simulink model "quad_mpc_nn_3_ref"  (R2020a)
settings: Solver=FixedStepAuto  StartTime=0.0  StopTime=20  FixedStep=0.01  RelTol=1e-3
values from neighbouring files (symbols this model uses):
  no_y = 6    [main_quad_mpc.m]
  x0 = [7;-10;0;0;0;0;0;0;0;0;0;0]    [main_quad_mpc.m]
libraries: neural x38
(part 3 of 3)

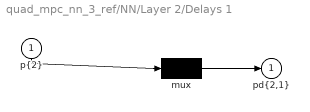
== system quad_mpc_nn_3_ref/NN/Layer 2/Delays 1 ==
  "p{2}" : Inport  PortDimensions=30
      mask Display: e = 0.06;c1 = [120 230 180]/255;c2 = ([120 230 180]+0)/(256+128);c3 = ([120 230 180]+128)/(256+128);patch([0 1 1 0],[0 0 1 1],c1);patch([0 1 1 1-e 1-e 0+e],[0 0 1 1-e 0+e 0+e],c2);patch([0 0 1 1-e 0+e 0+e],[0 1 1 1-e 1-e 0+e],c3);plot([0 1 1 0 0],[0 0 1 1 0]);
  mux : Mux  Inputs=1
      mask Display: e = 0.06;c1 = [120 150 230]/255;c2 = ([120 150 230]+0)/383;c3 = ([120 150 230]+128)/383;patch([0 1 1 0],[0 0 1 1],c1);patch([0 1 1 1-e 1-e 0+e],[0 0 1 1-e 0+e 0+e],c2);patch([0 0 1 1-e 0+e 0+e],[0 1 1 1-e 1-e 0+e],c3);plot([0 1 1 0 0],[0 0 1 1 0]);disp('Mux')
  "pd{2,1}" : Outport
      mask Display: e = 0.06;c1 = [120 230 180]/255;c2 = ([120 230 180]+0)/(256+128);c3 = ([120 230 180]+128)/(256+128);patch([0 1 1 0],[0 0 1 1],c1);patch([0 1 1 1-e 1-e 0+e],[0 0 1 1-e 0+e 0+e],c2);patch([0 0 1 1-e 0+e 0+e],[0 1 1 1-e 1-e 0+e],c3);plot([0 1 1 0 0],[0 0 1 1 0]);
  wires:
  "p{2}"/1 -> mux/1
  mux/1 -> "pd{2,1}"/1

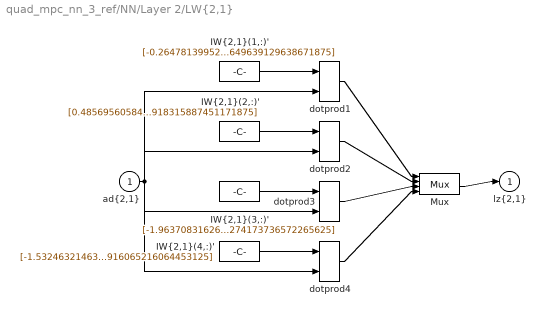
== system quad_mpc_nn_3_ref/NN/Layer 2/LW{2,1} ==
  "ad{2,1}" : Inport  PortDimensions=30
      mask Display: e = 0.06;c1 = [120 230 180]/255;c2 = ([120 230 180]+0)/(256+128);c3 = ([120 230 180]+128)/(256+128);patch([0 1 1 0],[0 0 1 1],c1);patch([0 1 1 1-e 1-e 0+e],[0 0 1 1-e 0+e 0+e],c2);patch([0 0 1 1-e 0+e 0+e],[0 1 1 1-e 1-e 0+e],c3);plot([0 1 1 0 0],[0 0 1 1 0]);
  "IW{2,1}(1,:)'" : Constant  Value=[-0.264781399520385096746366571096586994826793670654296875;-0.60161514587966891109971356854657642543315887451171875;0.034180266739349207671949670839239843189716339111328125;-0.545987433505061847682782172341831028461456298828125;2.979819360304903685943145319470204412937164306640625;0.77721513496705119106167103382176719605922698974609375;0.88667437951173033727769734468893148005008697509765625;-0.151868687305941885146154390895389951765537261962890625;-0.89945621880234838396717123032431118190288543701171875;0.315274650711938608793616367620415985584259033203125;-0.339046618347827621864354341596481390297412872314453125;-0.5901640579711642242699554117280058562755584716796875;0.408041226695667946788859126172610558569431304931640625;0.4516333770263789570975632159388624131679534912109375;-0.3872383159231318483506356642465107142925262451171875;0.32104169696543116696574315938050858676433563232421875;-1.1008051516787868973068498235079459846019744873046875;-0.03423394212066994957144316913399961777031421661376953125;0.2378870241662367213120177211749251000583171844482421875;0.3938028226142582521873691803193651139736175537109375;0.433952959579377850474202205077745020389556884765625;0.989524958311408742162029739120043814182281494140625;-0.14069682180978981822505602394812740385532379150390625;-0.0037746954761124495991708727160585112869739532470703125;-0.2174468074086713664794245914890780113637447357177734375;-0.037951766990621138564421244154800660908222198486328125;0.62177684299741520224102941938326694071292877197265625;0.8875905040341243168455775958136655390262603759765625;0.8521323346364033657351910733268596231937408447265625;-1.9734512621785114117045623061130754649639129638671875]
      mask Display: e = 0.06;c1 = [120 150 230]/255;c2 = ([120 150 230]+0)/383;c3 = ([120 150 230]+128)/383;patch([0 1 1 0],[0 0 1 1],c1);patch([0 1 1 1-e 1-e 0+e],[0 0 1 1-e 0+e 0+e],c2);patch([0 0 1 1-e 0+e 0+e],[0 1 1 1-e 1-e 0+e],c3);plot([0 1 1 0 0],[0 0 1 1 0]);disp('weights');
  "IW{2,1}(2,:)'" : Constant  Value=[0.48569560584269166891857594237080775201320648193359375;-1.3313184389286047970557547159842215478420257568359375;0.480486462600825892099720704209175892174243927001953125;1.17660400430466349774860645993612706661224365234375;2.01103395513448734988060095929540693759918212890625;0.51668028139238486584616794061730615794658660888671875;-0.28605587577639324248224284019670449197292327880859375;-1.98222942171470695171819897950626909732818603515625;-0.0215173953226786458803321266941566136665642261505126953125;-0.5618542526154275407179738976992666721343994140625;-2.295259765211787428285106216208077967166900634765625;0.2170034096592754480070652789436280727386474609375;-0.02018749857042749507041179413135978393256664276123046875;1.7472615771880792845394125833990983664989471435546875;-1.4166115970212143082562761264853179454803466796875;0.64044058881881171796379703664570115506649017333984375;1.3885358314738542873101323493756353855133056640625;0.9082194581400955257777241058647632598876953125;-0.45862032270002661693553136501577682793140411376953125;0.76901111434985358616955863908515311777591705322265625;-0.2764761886301432269874567282386124134063720703125;-0.311728394721483892393365522366366349160671234130859375;-0.06471671380954514829486612370601505972445011138916015625;-1.1918719761821898739384550935938023030757904052734375;-0.386339353922815875730378820662735961377620697021484375;-0.883222695234621379967165921698324382305145263671875;1.2122908779750136698538653945433907210826873779296875;1.1092779253445852472026444957009516656398773193359375;0.708487614769847340312480810098350048065185546875;0.307210640063644901953665566907147876918315887451171875]
      mask Display: e = 0.06;c1 = [120 150 230]/255;c2 = ([120 150 230]+0)/383;c3 = ([120 150 230]+128)/383;patch([0 1 1 0],[0 0 1 1],c1);patch([0 1 1 1-e 1-e 0+e],[0 0 1 1-e 0+e 0+e],c2);patch([0 0 1 1-e 0+e 0+e],[0 1 1 1-e 1-e 0+e],c3);plot([0 1 1 0 0],[0 0 1 1 0]);disp('weights');
  "IW{2,1}(3,:)'" : Constant  Value=[-1.96370831626150721405110743944533169269561767578125;0.1657688265350187595270625706689315848052501678466796875;-1.6700000677074264832100425337557680904865264892578125;-0.5144365955387382172148136305622756481170654296875;1.184422671048634523316422928473912179470062255859375;0.898253447640056545964171164087019860744476318359375;1.173662715707431747347300188266672194004058837890625;-1.0861297901202819904398211292573250830173492431640625;-0.009160020387555319054673219625328783877193927764892578125;-2.905483524807892958818911210983060300350189208984375;-0.248638304117494934875054468648158945143222808837890625;1.2234030220932023969027113707852549850940704345703125;-1.2964279816399650879787941448739729821681976318359375;0.165499461543745340907918262018938548862934112548828125;-1.6701128874882869013163144700229167938232421875;1.0539302091185105414439249216229654848575592041015625;0.624705280228390780195013576303608715534210205078125;-1.0064413728805312597813781394506804645061492919921875;-0.1566022648618327905989389137175749056041240692138671875;-1.3202191260088078639256536916946060955524444580078125;1.143794782413694033351703183143399655818939208984375;-1.507596235822215913202626325073651969432830810546875;0.203093685527490908082626219766098074615001678466796875;-1.1119097279994980542738858275697566568851470947265625;0.91117452076927840654008150522713549435138702392578125;-0.88823613654887345614241667135502211749553680419921875;-0.262623620221561215881678208461380563676357269287109375;1.053060557655885798311601320165209472179412841796875;-1.8537111295778085917618227540515363216400146484375;-2.326326843262569443737675101147033274173736572265625]
      mask Display: e = 0.06;c1 = [120 150 230]/255;c2 = ([120 150 230]+0)/383;c3 = ([120 150 230]+128)/383;patch([0 1 1 0],[0 0 1 1],c1);patch([0 1 1 1-e 1-e 0+e],[0 0 1 1-e 0+e 0+e],c2);patch([0 0 1 1-e 0+e 0+e],[0 1 1 1-e 1-e 0+e],c3);plot([0 1 1 0 0],[0 0 1 1 0]);disp('weights');
  "IW{2,1}(4,:)'" : Constant  Value=[-1.5324632146358980744338396107195876538753509521484375;-1.6845276501195958207546254925546236336231231689453125;-1.16884199275598188449976078118197619915008544921875;0.373180066038573177156223437123117037117481231689453125;0.1717742493880567433706119118141941726207733154296875;1.6840008258698169196776461831177584826946258544921875;1.0476154481897055337213942038943059742450714111328125;-0.02411712696231184394068947085543186403810977935791015625;-2.0031542278967133796641064691357314586639404296875;-0.92906759089245116722821649091201834380626678466796875;1.5331972741214590083558277910924516618251800537109375;1.237944294397044675548613668070174753665924072265625;-0.81887779466048582488468809970072470605373382568359375;-0.520342281881557511269420501776039600372314453125;0.833514714888559549166302531375549733638763427734375;2.171474819472868578174029607907868921756744384765625;-0.0828367864161536349154602021371829323470592498779296875;-0.55144091275721063283299372415058314800262451171875;1.097529366365379122072454265435226261615753173828125;-0.716082961678606633171284556738100945949554443359375;-1.294600018706635768950263809529133141040802001953125;-0.74288610068922178442107906448654830455780029296875;-0.9277758234567430317696334896027110517024993896484375;-0.1382620257497986504535703033980098553001880645751953125;0.903097685412288075923470387351699173450469970703125;0.7411215602549463543624597150483168661594390869140625;-0.7047838046634680164714836791972629725933074951171875;-1.6134564939277371564685381599701941013336181640625;1.02870679264472375535888204467482864856719970703125;0.613440194095904889337589338538236916065216064453125]
      mask Display: e = 0.06;c1 = [120 150 230]/255;c2 = ([120 150 230]+0)/383;c3 = ([120 150 230]+128)/383;patch([0 1 1 0],[0 0 1 1],c1);patch([0 1 1 1-e 1-e 0+e],[0 0 1 1-e 0+e 0+e],c2);patch([0 0 1 1-e 0+e 0+e],[0 1 1 1-e 1-e 0+e],c3);plot([0 1 1 0 0],[0 0 1 1 0]);disp('weights');
  Mux : Mux
      mask Display: e = 0.06;c1 = [120 150 230]/255;c2 = ([120 150 230]+0)/383;c3 = ([120 150 230]+128)/383;patch([0 1 1 0],[0 0 1 1],c1);patch([0 1 1 1-e 1-e 0+e],[0 0 1 1-e 0+e 0+e],c2);patch([0 0 1 1-e 0+e 0+e],[0 1 1 1-e 1-e 0+e],c3);plot([0 1 1 0 0],[0 0 1 1 0]);disp('Mux');
  dotprod{1..4} (4 alike) : neural/Weight Functions/dotprod
  "lz{2,1}" : Outport
      mask Display: e = 0.06;c1 = [120 230 180]/255;c2 = ([120 230 180]+0)/(256+128);c3 = ([120 230 180]+128)/(256+128);patch([0 1 1 0],[0 0 1 1],c1);patch([0 1 1 1-e 1-e 0+e],[0 0 1 1-e 0+e 0+e],c2);patch([0 0 1 1-e 0+e 0+e],[0 1 1 1-e 1-e 0+e],c3);plot([0 1 1 0 0],[0 0 1 1 0]);
  wires:
  "IW{2,1}(1,:)'"/1 -> dotprod1/1
  "ad{2,1}"/1 -> dotprod1/2, dotprod2/2, dotprod3/2, dotprod4/2
  dotprod1/1 -> Mux/1
  "IW{2,1}(2,:)'"/1 -> dotprod2/1
  dotprod2/1 -> Mux/2
  "IW{2,1}(3,:)'"/1 -> dotprod3/1
  dotprod3/1 -> Mux/3
  "IW{2,1}(4,:)'"/1 -> dotprod4/1
  dotprod4/1 -> Mux/4
  Mux/1 -> "lz{2,1}"/1
